simulink model "bclashtest"  (Simulink 8.3)
settings: Solver=ode5  SolverMode=SingleTasking  StartTime=0.0  StopTime=40  FixedStep=0.01  RelTol=1e-3  AbsTol=1e-6
settings Model: Creator=ikko  LastModifiedBy=ikko
settings DataIOCC: LimitDataPoints=off  SignalLoggingName=logsOut
settings OptimizationCC: BooleanDataType=off  ExpressionDepthLimit=2147483647  InitFltsAndDblsToZero=on
settings DebuggingCC: SaveWithParameterizedLinksMsg=none  CheckExecutionContextPreStartOutputMsg=on  CheckExecutionContextRuntimeOutputMsg=on  SignalResolutionControl=TryResolveAllWithWarning  SolverPrmCheckMsg=none  InheritedTsInSrcMsg=none  MultiTaskDSMMsg=warning  MultiTaskCondExecSysMsg=none  FcnCallInpInsideContextMsg=EnableAllAsWarning  StrictBusMsg=None
settings HardwareCC: TargetUnknown=on
settings RTWCC: TemplateMakefile=grt_vc.tmf  IncludeERTFirstTime=on
settings GRTTargetCC: TargetFcnLib=ansi_tfl_tmw.mat

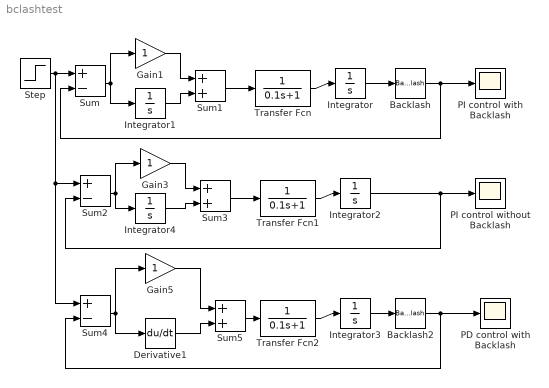
== system bclashtest ==
  Backlash : Backlash  BacklashWidth=0.5
  Backlash2 : Backlash  BacklashWidth=0.5
  Derivative1 : Derivative
  Gain1 : Gain  SaturateOnIntegerOverflow=on  OutDataTypeStr=Inherit: Same as input  ParamDataTypeStr=Inherit: Same as input
  Gain3 : Gain  SaturateOnIntegerOverflow=on  OutDataTypeStr=Inherit: Same as input  ParamDataTypeStr=Inherit: Same as input
  Gain5 : Gain  SaturateOnIntegerOverflow=on  OutDataTypeStr=Inherit: Same as input  ParamDataTypeStr=Inherit: Same as input
  Integrator{,1..4} (5 alike) : Integrator
  PD control with Backlash : Scope
      settings: TickLabels=on  YMin=0  YMax=8
  PI control with Backlash : Scope
      settings: TickLabels=on  YMin=0  YMax=8
  PI control without Backlash : Scope
      settings: TickLabels=on  YMin=0  YMax=8
  Step : Step  After=3
  Sum : Sum  Inputs=+-  SaturateOnIntegerOverflow=on  InputSameDT=on  OutDataTypeStr=Inherit: Same as first input
  Sum1 : Sum  SaturateOnIntegerOverflow=on  InputSameDT=on  OutDataTypeStr=Inherit: Same as first input
  Sum2 : Sum  Inputs=+-  SaturateOnIntegerOverflow=on  InputSameDT=on  OutDataTypeStr=Inherit: Same as first input
  Sum3 : Sum  SaturateOnIntegerOverflow=on  InputSameDT=on  OutDataTypeStr=Inherit: Same as first input
  Sum4 : Sum  Inputs=+-  SaturateOnIntegerOverflow=on  InputSameDT=on  OutDataTypeStr=Inherit: Same as first input
  Sum5 : Sum  SaturateOnIntegerOverflow=on  InputSameDT=on  OutDataTypeStr=Inherit: Same as first input
  Transfer Fcn : TransferFcn  Denominator=[0.1 1]
  Transfer Fcn1 : TransferFcn  Denominator=[0.1 1]
  Transfer Fcn2 : TransferFcn  Denominator=[0.1 1]
  wires:
  Derivative1/1 -> Sum5/2
  Integrator3/1 -> Backlash2/1
  Integrator2/1 -> PI control without Backlash/1, Sum2/2
  Integrator/1 -> Backlash/1
  Sum5/1 -> Transfer Fcn2/1
  Gain5/1 -> Sum5/1
  Backlash2/1 -> PD control with Backlash/1, Sum4/2
  Transfer Fcn2/1 -> Integrator3/1
  Sum4/1 -> Derivative1/1, Gain5/1
  Sum3/1 -> Transfer Fcn1/1
  Integrator4/1 -> Sum3/2
  Gain3/1 -> Sum3/1
  Transfer Fcn1/1 -> Integrator2/1
  Sum2/1 -> Integrator4/1, Gain3/1
  Step/1 -> Sum4/1, Sum2/1, Sum/1
  Sum1/1 -> Transfer Fcn/1
  Integrator1/1 -> Sum1/2
  Gain1/1 -> Sum1/1
  Backlash/1 -> PI control with Backlash/1, Sum/2
  Transfer Fcn/1 -> Integrator/1
  Sum/1 -> Integrator1/1, Gain1/1
